simulink model "scdintegerdelay"  (Simulink 7.6)
settings: Solver=VariableStepDiscrete  StartTime=0.0  StopTime=10.0  RelTol=1e-3
libraries: simulink x1
settings Model: Creator=The MathWorks Inc.
settings OptimizationCC: InitFltsAndDblsToZero=on
settings DebuggingCC: StrictBusMsg=Warning

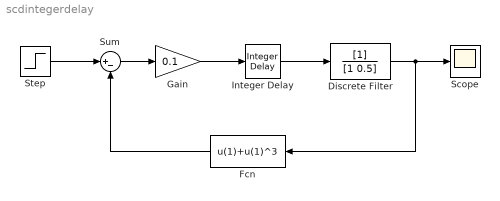
== system scdintegerdelay ==
  Discrete Filter : DiscreteFilter  SampleTime=0.01
  Fcn : Fcn  Expr=u(1)+u(1)^3
  Gain : Gain  Gain=0.1
  Integer Delay : simulink/Discrete/Integer Delay  NumDelays=20  InputProcessing=Inherited  vinit=0.0  samptime=0.01
  Scope : Scope
  Step : Step  SampleTime=0
  Sum : Sum  Inputs=|+-
  wires:
  Integer Delay/1 -> Discrete Filter/1
  Gain/1 -> Integer Delay/1
  Sum/1 -> Gain/1
  Discrete Filter/1 -> Scope/1, Fcn/1
  Step/1 -> Sum/1
  Fcn/1 -> Sum/2
